simulink library "dspobslib"  (Simulink 8.0)
settings: Solver=ode45  SolverMode=SingleTasking  StartTime=0.0  StopTime=10.0  RelTol=1e-3
values from neighbouring files (symbols this model uses):
  D = D + B    [rebuffer_delay.m]
  ic = eval(icStr)    [dsparch3Transform.m]
undefined symbols (not defined in the file or in its folder): phh, phl
libraries: dspsigattribs x14, dspsigops x5, dspobslib x3, dspmtrx3 x1, dspmathops x1, dspbuff3 x1
settings Model: RequirementInfo=9  Creator=don  LastModifiedBy=amoyer  CovMetricSettings=d  ExtModeAutoUpdateStatusClock=off
settings Model: ForwardingTableString=|
  | ||__slOldName__||dspobslib/Yule-Walker IIR
  | Filter Design||__slNewName__||dspddes3/Yule-Walker IIR
  | Filter Design||__slOldName__||dspobslib/Digital IIR
  | Filter Design||__slNewName__||dspddes3/Digital IIR
  | Filter Design||__slOldName__||dspobslib/Digital FIR Raised
  | Cosine Filter Design||__slNewName__||dspddes3/Digital FIR Raised
  | Cosine Filter Design||__slOldName__||dspobslib/Least Squares FIR
  | Filter Design||__slNewName__||dspddes3/Least Squares FIR
  | Filter Design||__slOldName__||dspobslib/Remez FIR
  | Filter Design||__slNewName__||dspddes3/Remez FIR
  | Filter Design||__slOldName__||dspobslib/Digital FIR
  | Filter Design||__slNewName__||dspddes3/Digital FIR
  | Filter Design||__slOldName__||dspobslib/Time-Varying
  | Lattice Filter||__slNewName__||dsparch3/Time-Varying
  | Lattice Filter||__slOldName__||dspobslib/Time-Varying Direct-
  | Form II Transpose Filter||__slNewName__||dsparch3/Time-Varying Direct-
  | Form II Transpose Filter||__slOldName__||dspobslib/Direct-Form II
  | Transpose Filter||__slNewName__||dsparch3/Direct-Form II
  | Transpose Filter||__slOldName__||dspobslib/Biquadratic
  | Filter||__slNewName__||dsparch4/Biquad Filter

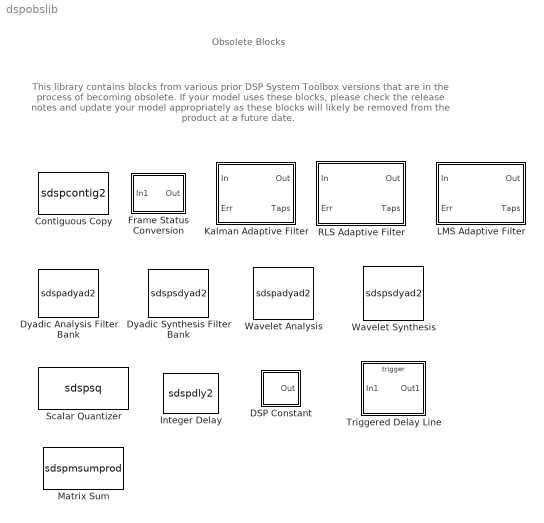
== system dspobslib ==
  note: Obsolete Blocks
  note: This library contains blocks from various prior DSP System Toolbox versions
      | that are in the process of becoming obsolete. If your model uses these blocks, please
      | check the release notes and update your model appropriately as these blocks will likely
      | be removed from the product at a future date.
  Contiguous Copy : S-Function  FunctionName=sdspcontig2  EnableBusSupport=off  mask(Contiguous Copy){}
      mask help: Create a contiguous copy of input data. For use with blocks that only accept contiguous data during simulation or code generation.
      mask Help: eval('blocksethelp');
      mask Display: disp('Contiguous\nCopy');
  DSP Constant : Subsystem  mask(DSP Constant){Value=1, SampleMode=Discrete, discreteOutput=Sample-based, continuousOutput=Sample-based, sampTime=1, framePeriod=2, additionalParams=off, allowOverrides=on, dataType=Inherit from 'Constant value', isSigned=on, wordLen=16, udDataType=sfix(16), fracBitsMode=Best precision, numFracBits=15, InterpretAs1D=-inf, Ts=-inf, FramebasedOutput=-inf}
      mask prompts: Value "Constant value:"; SampleMode "Sample mode:"; discreteOutput "Output:"; continuousOutput "Output:"; sampTime "Sample time:"; framePeriod "Frame period:"; additionalParams "------- Show additional parameters --------"; allowOverrides "Allow overrides from DSP Fixed-Point Attributes blocks"; dataType "Output data type:"; isSigned "Signed"; wordLen "Word length:"; udDataType "User-defined data type:"; fracBitsMode "Set fraction length in output to:"; numFracBits "Fraction length:"; InterpretAs1D "old Interpret as 1D checkbox"; Ts "old Sample time/Frame period"; FramebasedOutput "old Frame-based output checkbox"
      mask help: Output a discrete-time or continuous-time constant.
      mask init:
      | dispValue = get_param(gcbh, 'Value');
      | dspblkdspconst2('init');
      | dspblkdspconst2('update');
      mask Help: eval('blocksethelp');
      mask TypeOptions SampleMode: Discrete | Continuous
      mask Callback SampleMode: dspblkdspconst2;
      mask TypeOptions discreteOutput: Sample-based (interpret vectors as 1-D) | Sample-based | Frame-based
      mask Callback discreteOutput: dspblkdspconst2;
      mask TypeOptions continuousOutput: Sample-based (interpret vectors as 1-D) | Sample-based
      mask Callback continuousOutput: dspblkdspconst2;
      mask TypeOptions dataType: double | single | int8 | uint8 | int16 | uint16 | int32 | uint32 | boolean | Fixed-point | User-defined | Inherit from 'Constant value' | Inherit via back propagation
      mask Callback dataType: dspblkdspconst2;
      mask Callback udDataType: dspblkdspconst2;
      mask TypeOptions fracBitsMode: Best precision | User-defined
      mask Callback fracBitsMode: dspblkdspconst2;
      mask Display: disp(dispValue);
  Dyadic Analysis Filter Bank : S-Function  FunctionName=sdspadyad2  Parameters=phl,phh,numLevels,tree, hl, hh  EnableBusSupport=off  mask(Dyadic Analysis Filter Bank){hl=fir1(12,0.4), hh=fir1(12,0.6,'high'), numLevels=2, tree=Asymmetric}
      mask prompts: hl "Lowpass FIR filter coefficients:"; hh "Highpass FIR filter coefficients:"; numLevels "Number of levels:"; tree "Tree structure:"
      mask help: Apply a sequence of FIR filters to the input signal, downsampling by two following each filtering operation. With reference to the icon on the block, a lowpass filter is applied at each descending branch and a highpass filter is applied at each non-descending branch. Normally, the lowpass and highpass filters are complementary, as in a typical wavelet-based signal decomposition.
      mask init:
      | [phl,phh,x,y,str] = dspblkadyad2(hl,hh,numLevels,tree);
      mask Help: eval('blocksethelp');
      mask TypeOptions tree: Asymmetric | Symmetric
      mask Display:
      | text(0.1,0.15,str)
      | plot(x,y)
  Dyadic Synthesis Filter Bank : S-Function  FunctionName=sdspsdyad2  Parameters=phl,phh,numLevels,tree,hl,hh  EnableBusSupport=off  mask(Dyadic Synthesis Filter Bank){hl=fir1(12,0.4), hh=fir1(12,0.6,'high'), numLevels=2, tree=Asymmetric}
      mask prompts: hl "Lowpass FIR filter coefficients:"; hh "Highpass FIR filter coefficients:"; numLevels "Number of levels:"; tree "Tree structure:"
      mask help: Apply a sequence of FIR filters to the input signals, upsampling by two following each filtering operation. With reference to the icon on the block, a lowpass filter is applied at each descending branch and a highpass filter is applied at each non-descending branch. Normally, the lowpass and highpass filters are complementary, as in a typical wavelet-based signal reconstruction.
      mask init:
      | [phl,phh,x,y,str] = dspblksdyad2(hl,hh,numLevels,tree);
      mask Help: eval('blocksethelp');
      mask TypeOptions tree: Asymmetric | Symmetric
      mask Display:
      | text(0.80,0.15,str)
      | plot(x,y)
  Frame Status Conversion : Subsystem  mask(Frame Status Conversion){growRefPort=off, outframe=Frame-based}
      mask prompts: growRefPort "Inherit output frame status from Ref input port"; outframe "Output signal:"
      mask help: Specify the frame status of the output signal.
      mask init:
      | [p, str] = dspblkfrmconv('init');
      mask Help: eval('blocksethelp');
      mask Callback growRefPort: dspblkfrmconv
      mask TypeOptions outframe: Frame-based | Sample-based
      mask Display:
      | port_label(p.in1,   p.i1,  p.i1s);
      | port_label(p.in2,   p.i2,  p.i2s);
      | port_label(p.out, p.o1, p.o1s);
      | disp(str)
  Integer Delay : S-Function  FunctionName=sdspdly2  Parameters=delay,ic,reset  EnableBusSupport=off  mask(Integer Delay){delay=1, ic=0, reset_popup=None}
      mask prompts: delay "Delay (samples):"; ic "Initial conditions:"; reset_popup "Reset port:"
      mask help: Delay discrete-time input by a fixed integer number of sample periods.
      mask init:
      | delayValue = get_param(gcbh, 'delay');
      | str = dspblkdly2('icon',delayValue,delay);
      | dx = 0.01*length(str);
      | reset = reset_popup-1;
      | if (reset == 0)
      | 	s.i1 = 1; s.i1s = '';
      | 	s.i2 = 1; s.i2s = '';
      | else
      | 	s.i1 = 1; s.i1s = 'In';
      | 	s.i2 = 2; s.i2s = 'Rst';
      | end
      mask Help: eval('blocksethelp');
      mask TypeOptions reset_popup: None | Rising edge | Falling edge | Either edge | Non-zero sample
      mask Display:
      | text(0.42-dx, 0.4, 'z'); text(0.5-dx, 0.6, str);
      | port_label('input',s.i1,s.i1s);
      | port_label('input',s.i2,s.i2s);
  Kalman Adaptive Filter : Subsystem  mask(Kalman Adaptive Filter){Ntaps=64, Jmin=0.3, q=0.1, ic0=0, K0=0.5, Adapt=off, RstPort=None}
      mask prompts: Ntaps "FIR filter length:"; Jmin "Measurement noise variance:"; q "Process noise variance:"; ic0 "Initial value of filter taps:"; K0 "Initial error correlation matrix:"; Adapt "Adapt port"; RstPort "Reset port:"
      mask help:
      | One-step Kalman predictor algorithm for adaptive FIR filtering of input signal.
      |
      | Select the Adapt port check box to create an Adapt port on the block. When the input to this port is nonzero, the block enables filter adaptation. When the input to this port is zero, filter adaptation is disabled.
      |
      | If the Reset port is enabled and a reset event occurs, the block resets the filter weights to their initial values.
      mask init:
      | if prod(size(ic0))==1, ic = ic0(ones(Ntaps,1)); else ic = ic0; end
      | if prod(size(K0))==1, K = K0.*eye(Ntaps);
      | elseif any(size(K0)==1), K = diag(K0);
      | else K=K0; end
      | % ic = ic0;
      | % K = K0;
      | dspblkadpt('init');
      mask Help: eval('blocksethelp');
      mask TypeOptions RstPort: None | Rising edge | Falling edge | Either edge | Non-zero sample
      mask Display: disp('Kalman')
  LMS Adaptive Filter : Subsystem  mask(LMS Adaptive Filter){n=32, mu=.65, ic=0.0, leakage=1.0, normalized=on, Adapt=off, RstPort=None}
      mask prompts: n "FIR filter length:"; mu "Step-size, mu:"; ic "Initial value of filter taps:"; leakage "Leakage factor (0 to 1):"; normalized "Use normalization"; Adapt "Adapt input"; RstPort "Reset input:"
      mask help:
      | Least mean-square (LMS) algorithm for adaptive FIR filtering of input signal.  Energy normalization may optionally be disabled.
      |
      | If 'Adapt input' is checked and the Adapt signal is zero, the algorithm temporarily disables adaptation of the filter coefficients.  A non-zero signal enables filter adaptation.
      |
      | If the 'Reset input' is enabled and the Reset signal transitions appropriately, the filter coefficients are reset to the initial conditions.
      mask init:
      | if normalized, s='nLMS'; else s='LMS'; end
      | dspblkadpt('init');
      mask Help: eval('blocksethelp');
      mask TypeOptions RstPort: None | Rising edge | Falling edge | Either edge | Non-zero sample
      mask Display: disp(s);
  Matrix Sum : S-Function  DialogController=dspDDGCreate  DialogControllerArgs=DataTag3  FunctionName=sdspmsumprod  Parameters=Dim,1,[],[],-1,0,0,-1,0,0,dtInfo.accumMode,dtInfo.accumWordLength,dtInfo.accumFracLength,dtInfo.outputMode,dtInfo.outputWordLength,dtInfo.outputFracLength,dtInfo.roundingMode,dtInfo.overflowMode  EnableBusSupport=off  mask(Matrix Sum){Dim=Columns, additionalParams=off, allowOverrides=on, outputMode=Same as accumulator, outputWordLength=16, outputFracLength=15, accumMode=Inherit via internal rule, accumWordLength=32, accumFracLength=30, roundingMode=Floor, overflowMode=off, LockScale=off}
      mask prompts: Dim "Sum over:"; additionalParams "------- Show additional parameters -------"; allowOverrides "Allow overrides from DSP Fixed-Point Attributes blocks"; outputMode "Fixed-point output attributes:"; outputWordLength "Output word length:"; outputFracLength "Output fraction length:"; accumMode "Fixed-point accumulator attributes:"; accumWordLength "Accumulator word length:"; accumFracLength "Accumulator fraction length:"; roundingMode "Round integer calculations toward:"; overflowMode "Saturate on integer overflow"; LockScale "Lock scaling"
      mask help: Sum the elements of a matrix along its rows, its columns, or over all its elements. Note that 1-D input signals produce a single scalar output equal to the sum of the individual elements.
      mask init:
      | if (Dim==1), str='Row\nSum';
      | elseif (Dim==2), str='Column\nSum';
      | else str='Sum of\nAll Elements';
      | end
      | 
      | %misc       1 USED
      | %output     2 USED
      | %accum      4 USED
      | dtInfo = dspGetFixptDataTypeInfo(gcbh,7);
      mask Help: eval('blocksethelp');
      mask TypeOptions Dim: Rows | Columns | Entire input
      mask TypeOptions outputMode: Same as accumulator | Same as input | Binary point scaling | Slope and bias scaling | User-defined
      mask TypeOptions accumMode: Inherit via internal rule | Same as input | Binary point scaling | Slope and bias scaling | User-defined
      mask TypeOptions roundingMode: Ceiling | Convergent | Floor | Nearest | Round | Simplest | Zero
      mask Display: disp(str);
  RLS Adaptive Filter : Subsystem  mask(RLS Adaptive Filter){Ntaps=32, Lambda=1.0, ic=0.0, phi0=0.1, Adapt=off, RstPort=None}
      mask prompts: Ntaps "FIR filter length:"; Lambda "Memory weighting factor (0 to 1):"; ic "Initial value of filter taps:"; phi0 "Initial input variance estimate:"; Adapt "Adapt input"; RstPort "Reset input:"
      mask help:
      | Exponentially weighted recursive least-squares (RLS) algorithm for adaptive FIR filtering of input signal.
      |
      | If 'Adapt input' is checked and the Adapt signal is zero, the algorithm temporarily disables adaptation of the filter coefficients.  A non-zero signal enables filter adaptation.
      |
      | If the 'Reset input' is enabled and the Reset signal transitions appropriately, the filter coefficients are reset to the initial conditions.
      mask init:
      | dspblkadpt('init');
      mask Help: eval('blocksethelp');
      mask TypeOptions RstPort: None | Rising edge | Falling edge | Either edge | Non-zero sample
      mask Display: disp('RLS')
  Scalar Quantizer : S-Function  FunctionName=sdspsq  Parameters=Qmode,QparamSource,partitionUnBound,codebook,SearchMethod,tieBreakRule,outQError, invalidin, dtype, idtype, cwdtype,1,1  EnableBusSupport=off  mask(Scalar Quantizer){Qmode=Encoder, QparamSource=Specify via dialog, partitionUnBound=[   0  1  2  3  4  5    6  7  8    9], codebook=[0.0    1.5     2.5    3.5    4.5   5.5   6.5  7.5  8.5 ], SearchMethod=Binary, tieBreakRule=Choose the lower index, outQError=off, invalidin=Clip and warn, dtype=off, idtype=int32, cwdtype=double}
      mask prompts: Qmode "Quantizer mode:"; QparamSource "Source of quantizer parameters:"; partitionUnBound "Boundary points:"; SearchMethod "Searching method:"; tieBreakRule "Tie-breaking rule:"; outQError "Output the quantization error"; invalidin "Action for out of range input:"; dtype "--------------- Show additional parameters ---------------"; idtype "Output index data type:"; cwdtype "Output data type:"
      mask help:
      | The Scalar Quantizer block has three modes of operation.
      | In Encoder mode, the block maps each input value to a quantization region by comparing the input value to the user-specified quantizer boundary points. The block outputs the index of the associated region.
      | In Decoder mode, the block transforms the input index values into quantized output values, defined by the quantizer codebook.
      | In the Encoder & Decoder mode, the block performs both the encoding and decoding operations. The block outputs the index values and the quantized output values.
      |
      | The Boundary points parameter is a vector of dimension N whose values are arranged in ascending order ([p1 p2 ... pN]). The quantizer codebook is a vector of length (N-1). The quantizer is unbounded if p1 is -inf and pN is inf. When the quantizer is bounded, p1 is the lower bound for the input values. Any input less than p1 is clipped to p1 and then quantized. Similarly, pN is the upper bound for the input values. Any input greater than pN is clipped to pN and is then quantized.
      mask init:
      | [si,so,disp_str]=dspblksq('icon');
      mask Help: eval('blocksethelp');
      mask TypeOptions Qmode: Encoder | Decoder | Encoder and decoder
      mask Callback Qmode: dspblksq
      mask TypeOptions QparamSource: Specify via dialog | Input ports
      mask Callback QparamSource: dspblksq
      mask TypeOptions SearchMethod: Linear | Binary
      mask TypeOptions tieBreakRule: Choose the lower index | Choose the higher index
      mask TypeOptions invalidin: Clip | Clip and warn | Error
      mask Callback invalidin: dspblksq
      mask Callback dtype: dspblksq
      mask TypeOptions idtype: int8 | uint8 | int16 | uint16 | int32 | uint32
      mask TypeOptions cwdtype: double | single | int8 | uint8 | int16 | uint16 | int32 | uint32
      mask Display:
      | disp(disp_str);
      | port_label('input',si(1).port, si(1).txt);
      | port_label('input',si(2).port, si(2).txt);
      | port_label('input',si(3).port, si(3).txt);
      | port_label('output',so(1).port, so(1).txt);
      | port_label('output',so(2).port, so(2).txt);
      | port_label('output',so(3).port, so(3).txt);
  Triggered Delay Line : Subsystem  TreatAsAtomicUnit=on  mask(Triggered Delay Line){trig=Rising edge, siz=64, ic=0, TreatMby1Signals=One channel}
      mask prompts: trig "Trigger type:"; siz "Delay line size:"; ic "Initial conditions:"; TreatMby1Signals "Treat Mx1 and unoriented sample-based signals as:"
      mask help: Shift out delay line contents and store input data into start of delay line when trigger event occurs.
      mask init:
      | switch trig
      | case 1, s='rising';
      | case 2, s='falling';
      | case 3, s='either';
      | end
      | set_param([gcb '/Trigger'],'triggertype',s);
      | 
      | blkh = gcbh;
      | blkUserData = get_param(blkh, 'UserData');
      | if ~isfield(blkUserData, 'hasMChanOption')
      |     % Create and save the UserData field
      |     blkUserData.hasMChanOption = true;
      |     set_param(blkh, 'UserDataPersistent', 'on', ...
      |     'UserData', blkUserData);
      |     set_param(blkh, 'TreatMby1Signals', ...
      |     'M channels (this choice will be removed - see release notes)');
      | end
      | 
      | treat = get_param(blkh, 'TreatMby1Signals');
      | set_param([gcb '/Delay Line'], 'TreatMby1Signals', treat);
      mask Help: eval('blocksethelp');
      mask TypeOptions trig: Rising edge | Falling edge | Either edge
      mask TypeOptions TreatMby1Signals: One channel | M channels (this choice will be removed - see release notes)
      mask Display: disp('Delay\nLine');
  Wavelet Analysis : S-Function  FunctionName=sdspadyad2  Parameters=phl, phh, NumLevels, tree, hl, hh  EnableBusSupport=off  mask(Wavelet Analysis){Wname=Haar, OrdRec_ordDec=[1 / 1], Order=2, NumLevels=2}
      mask prompts: Wname "Wavelet name:"; OrdRec_ordDec "Filter order [synthesis / analysis]:"; Order "Wavelet order:"; NumLevels "Number of levels:"
      mask help:
      | Multilevel discrete 1-D wavelet decomposition using a specific wavelet.
      |
      | The Wavelet Toolbox must be installed to use this block.
      mask init:
      | [x,y,str] = dspblkwavedec2('icon');
      | [phl, phh, tree, hl, hh] = dspblkwavedec2('init');
      mask Help: eval('blocksethelp');
      mask TypeOptions Wname: Haar | Daubechies | Symlets | Coiflets | Biorthogonal | Reverse Biorthogonal | Discrete Meyer
      mask Callback Wname: dspblkwavedec2
      mask TypeOptions OrdRec_ordDec: [1 / 1] | [1 / 3] | [1 / 5] | [2 / 2] | [2 / 4] | [2 / 6] | [2 / 8] | [3 / 1] | [3 / 3] | [3 / 5] | [3 / 7] | [3 / 9] | [4 / 4] | [5 / 5] | [6 / 8]
      mask Display:
      | text(0.08,0.1,str)
      | plot(x,y)
  Wavelet Synthesis : S-Function  FunctionName=sdspsdyad2  Parameters=phl, phh, NumLevels, tree, hl, hh  EnableBusSupport=off  mask(Wavelet Synthesis){Wname=Haar, OrdRec_ordDec=[1 / 1], Order=2, NumLevels=2}
      mask prompts: Wname "Wavelet name:"; OrdRec_ordDec "Filter order [synthesis, analysis]:"; Order "Wavelet order:"; NumLevels "Number of levels:"
      mask help:
      | Multilevel discrete 1-D wavelet reconstruction using a specific wavelet.
      |
      | The Wavelet Toolbox must be installed to use this block.
      mask init:
      | [x,y,str] = dspblkwaverec2('icon');
      | [phl, phh, tree, hl, hh] = dspblkwaverec2('init');
      mask Help: eval('blocksethelp');
      mask TypeOptions Wname: Haar | Daubechies | Symlets | Coiflets | Biorthogonal | Reverse Biorthogonal | Discrete Meyer
      mask Callback Wname: dspblkwaverec2
      mask TypeOptions OrdRec_ordDec: [1 / 1] | [1 / 3] | [1 / 5] | [2 / 2] | [2 / 4] | [2 / 6] | [2 / 8] | [3 / 1] | [3 / 3] | [3 / 5] | [3 / 7] | [3 / 9] | [4 / 4] | [5 / 5] | [6 / 8]
      mask Display:
      | text(0.37,0.15,str)
      | plot(x,y)

== system dspobslib/DSP Constant ==
  Constant : Constant  Value=Value  VectorParams1D=off  SampleTime=sampTime
  Frame Status Conversion : FrameConversion  OutFrame=Sample-based
  Out : Outport
  wires:
  Constant/1 -> Frame Status Conversion/1
  Frame Status Conversion/1 -> Out/1

== system dspobslib/Frame Status Conversion ==
  In1 : Inport
  Frame Status : FrameConversion
  Out : Outport
  wires:
  In1/1 -> Frame Status/1
  Frame Status/1 -> Out/1

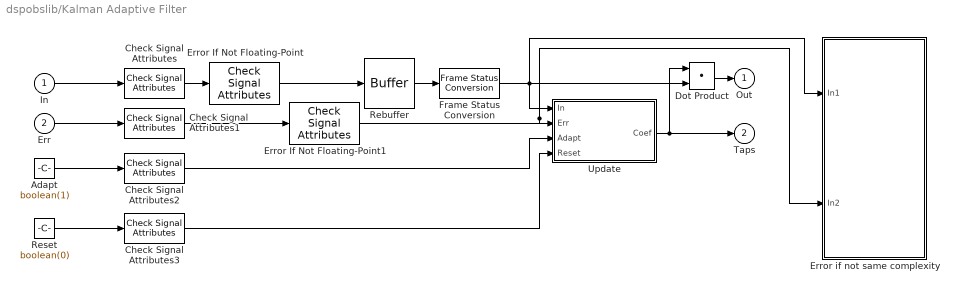
== system dspobslib/Kalman Adaptive Filter ==
  In : Inport
  Err : Inport  Port=2
  Adapt : Constant  Value=boolean(1)
  Check Signal Attributes{,1..3} (4 alike) : dspsigattribs/Check Signal Attributes  SystemSampleTime=-1  SigAttribCheckMethod=Does not match attributes exactly  Complexity=Ignore  Frame=Sample-based  DimsCheckMethod=Is...  Dimensions=Scalar (1-D or 2-D)  DatatypeCheckMethod=Ignore  DatatypeGeneral=Boolean  DtypeFloatSpecific=Any floating-point  DtypeFixedSpecific=Any fixed-point  DtypeIntSpecific=Any integer  SampleMode=Ignore
  Dot Product : DotProduct  OutDataTypeStr=Inherit: Inherit via internal rule
  Error If Not Floating-Point : dspsigattribs/Check Signal Attributes  SystemSampleTime=-1  SigAttribCheckMethod=Does not match attributes exactly  Complexity=Ignore  Frame=Ignore  DimsCheckMethod=Ignore  Dimensions=1-D  DatatypeCheckMethod=Is...  DatatypeGeneral=Floating-point  DtypeFloatSpecific=Any floating-point  DtypeFixedSpecific=Any fixed-point  DtypeIntSpecific=Any integer  SampleMode=Ignore
  Error If Not Floating-Point1 : dspsigattribs/Check Signal Attributes  SystemSampleTime=-1  SigAttribCheckMethod=Does not match attributes exactly  Complexity=Ignore  Frame=Ignore  DimsCheckMethod=Ignore  Dimensions=1-D  DatatypeCheckMethod=Is...  DatatypeGeneral=Floating-point  DtypeFloatSpecific=Any floating-point  DtypeFixedSpecific=Any fixed-point  DtypeIntSpecific=Any integer  SampleMode=Ignore
  Error if not same complexity : Subsystem  TreatAsAtomicUnit=on  SimViewingDevice=on
  Frame Status Conversion : dspobslib/Frame Status Conversion  SystemSampleTime=-1  growRefPort=off  outframe=Sample-based
  Rebuffer : Buffer  N=Ntaps  V=Ntaps-1  TreatMby1Signals=One channel
  Reset : Constant  Value=boolean(0)
  Update : Subsystem
  Out : Outport  InitialOutput=0
  Taps : Outport  Port=2  InitialOutput=0
  wires:
  Err/1 -> Check Signal Attributes1/1
  In/1 -> Check Signal Attributes/1
  Adapt/1 -> Check Signal Attributes2/1
  Dot Product/1 -> Out/1
  Rebuffer/1 -> Frame Status Conversion/1
  Update/1(Coef) -> Taps/1, Dot Product/1
  Check Signal Attributes1/1 -> Error If Not Floating-Point1/1
  Check Signal Attributes/1 -> Error If Not Floating-Point/1
  Check Signal Attributes2/1 -> Update/3(Adapt)
  Frame Status Conversion/1 -> Update/1(In), Dot Product/2, Error if not same complexity/1(In1)
  Reset/1 -> Check Signal Attributes3/1
  Check Signal Attributes3/1 -> Update/4(Reset)
  Error If Not Floating-Point/1 -> Rebuffer/1
  Error If Not Floating-Point1/1 -> Error if not same complexity/2(In2), Update/2(Err)

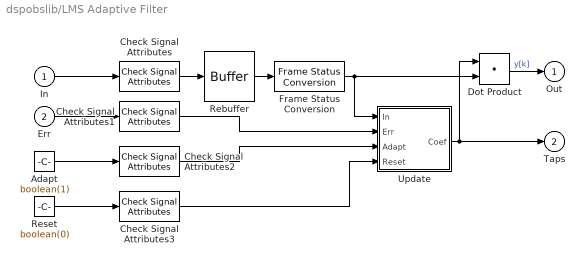
== system dspobslib/LMS Adaptive Filter ==
  In : Inport
  Err : Inport  Port=2
  Adapt : Constant  Value=boolean(1)
  Check Signal Attributes{,1..3} (4 alike) : dspsigattribs/Check Signal Attributes  SigAttribCheckMethod=Does not match attributes exactly  Complexity=Ignore  Frame=Sample-based  DimsCheckMethod=Is...  Dimensions=Scalar (1-D or 2-D)  DatatypeCheckMethod=Ignore  DatatypeGeneral=Boolean  DtypeFloatSpecific=Any floating-point  DtypeFixedSpecific=Any fixed-point  DtypeIntSpecific=Any integer  SampleMode=Ignore
  Dot Product : DotProduct  InputSameDT=on  OutDataTypeStr=Inherit: Inherit via internal rule
  Frame Status Conversion : dspobslib/Frame Status Conversion  growRefPort=off  outframe=Sample-based
  Rebuffer : Buffer  N=n  V=n-1  TreatMby1Signals=One channel
  Reset : Constant  Value=boolean(0)
  Update : Subsystem
  Out : Outport  InitialOutput=0
  Taps : Outport  Port=2  InitialOutput=0
  wires:
  Dot Product/1 -> Out/1  "y[k]"
  Update/1(Coef) -> Taps/1, Dot Product/1
  Rebuffer/1 -> Frame Status Conversion/1
  In/1 -> Check Signal Attributes/1
  Check Signal Attributes/1 -> Rebuffer/1
  Err/1 -> Check Signal Attributes1/1
  Check Signal Attributes1/1 -> Update/2(Err)
  Adapt/1 -> Check Signal Attributes2/1
  Check Signal Attributes2/1 -> Update/3(Adapt)
  Frame Status Conversion/1 -> Update/1(In), Dot Product/2
  Reset/1 -> Check Signal Attributes3/1
  Check Signal Attributes3/1 -> Update/4(Reset)

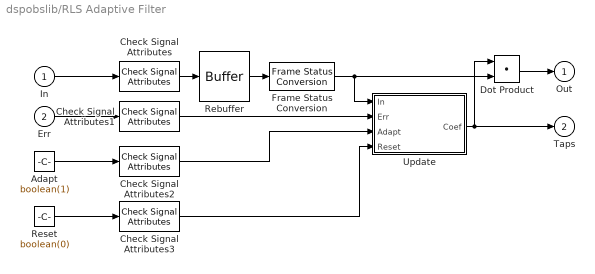
== system dspobslib/RLS Adaptive Filter ==
  In : Inport
  Err : Inport  Port=2
  Adapt : Constant  Value=boolean(1)
  Check Signal Attributes{,1..3} (4 alike) : dspsigattribs/Check Signal Attributes  SigAttribCheckMethod=Does not match attributes exactly  Complexity=Ignore  Frame=Sample-based  DimsCheckMethod=Is...  Dimensions=Scalar (1-D or 2-D)  DatatypeCheckMethod=Ignore  DatatypeGeneral=Boolean  DtypeFloatSpecific=Any floating-point  DtypeFixedSpecific=Any fixed-point  DtypeIntSpecific=Any integer  SampleMode=Ignore
  Dot Product : DotProduct  InputSameDT=on  OutDataTypeStr=Inherit: Inherit via internal rule
  Frame Status Conversion : dspobslib/Frame Status Conversion  growRefPort=off  outframe=Sample-based
  Rebuffer : Buffer  N=Ntaps  V=Ntaps-1  TreatMby1Signals=One channel
  Reset : Constant  Value=boolean(0)
  Update : Subsystem
  Out : Outport  InitialOutput=0
  Taps : Outport  Port=2  InitialOutput=0
  wires:
  Dot Product/1 -> Out/1
  Update/1(Coef) -> Taps/1, Dot Product/1
  Rebuffer/1 -> Frame Status Conversion/1
  In/1 -> Check Signal Attributes/1
  Check Signal Attributes/1 -> Rebuffer/1
  Err/1 -> Check Signal Attributes1/1
  Check Signal Attributes1/1 -> Update/2(Err)
  Adapt/1 -> Check Signal Attributes2/1
  Check Signal Attributes2/1 -> Update/3(Adapt)
  Frame Status Conversion/1 -> Update/1(In), Dot Product/2
  Reset/1 -> Check Signal Attributes3/1
  Check Signal Attributes3/1 -> Update/4(Reset)

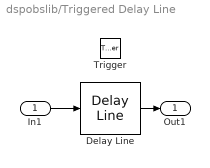
== system dspobslib/Triggered Delay Line ==
  In1 : Inport
  Trigger : TriggerPort  ZeroCross=off
  Delay Line : dspbuff3/Delay Line  siz=siz  ic=ic  directfeed=off  enable_output=off  hold_output=off  TreatMby1Signals=One channel
  Out1 : Outport  InitialOutput=ic
  wires:
  In1/1 -> Delay Line/1
  Delay Line/1 -> Out1/1

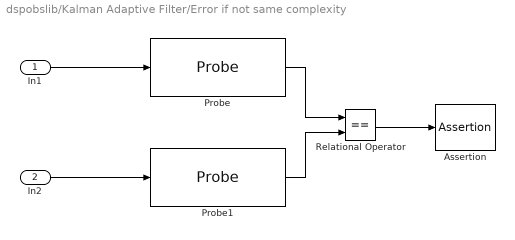
== system dspobslib/Kalman Adaptive Filter/Error if not same complexity ==
  In1 : Inport
  In2 : Inport  Port=2
  Assertion : Assertion  Enabled=on  AssertionFailFcn=error('The signals connected to the Input and Error ports of the Kalman Adaptive Filter block must have the same complexity.')
  Probe : Probe  ProbeWidth=off  ProbeSampleTime=off  ProbeComplexityDataType=boolean
  Probe1 : Probe  ProbeWidth=off  ProbeSampleTime=off  ProbeComplexityDataType=boolean
  Relational Operator : RelationalOperator  Operator===  OutDataTypeStr=boolean  ZeroCross=off  InputSameDT=on
  wires:
  Probe/1 -> Relational Operator/1
  Probe1/1 -> Relational Operator/2
  In1/1 -> Probe/1
  In2/1 -> Probe1/1
  Relational Operator/1 -> Assertion/1

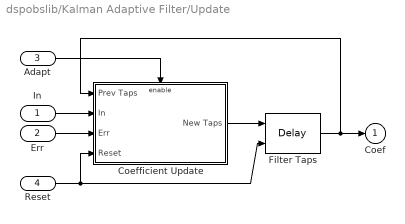
== system dspobslib/Kalman Adaptive Filter/Update ==
  In : Inport
  Err : Inport  Port=2
  Adapt : Inport  Port=3
  Reset : Inport  Port=4
  Coefficient Update : Subsystem  TreatAsAtomicUnit=on
  Filter Taps : dspsigops/Delay  dly_unit=Samples  delay=1  ic_detail=off  dif_ic_for_ch=on  dif_ic_for_dly=off  ic=ic  reset_popup=Non-zero sample
  Coef : Outport  InitialOutput=0
  wires:
  Filter Taps/1 -> Coef/1, Coefficient Update/1(Prev Taps)
  Coefficient Update/1(New Taps) -> Filter Taps/1
  In/1 -> Coefficient Update/2(In)
  Err/1 -> Coefficient Update/3(Err)
  Adapt/1 -> Coefficient Update/Enable
  Reset/1 -> Coefficient Update/4(Reset), Filter Taps/2

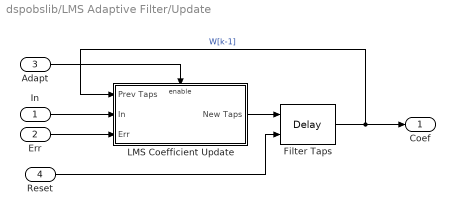
== system dspobslib/LMS Adaptive Filter/Update ==
  In : Inport
  Err : Inport  Port=2
  Adapt : Inport  Port=3
  Reset : Inport  Port=4
  Filter Taps : dspsigops/Delay  dly_unit=Samples  delay=1  ic_detail=off  dif_ic_for_ch=off  dif_ic_for_dly=off  ic=ic  reset_popup=Non-zero sample
  LMS Coefficient Update : Subsystem  TreatAsAtomicUnit=on
  Coef : Outport  InitialOutput=0
  wires:
  LMS Coefficient Update/1(New Taps) -> Filter Taps/1
  Err/1 -> LMS Coefficient Update/3(Err)
  In/1 -> LMS Coefficient Update/2(In)
  Filter Taps/1 -> Coef/1, LMS Coefficient Update/1(Prev Taps)  "W[k-1]"
  Adapt/1 -> LMS Coefficient Update/Enable
  Reset/1 -> Filter Taps/2

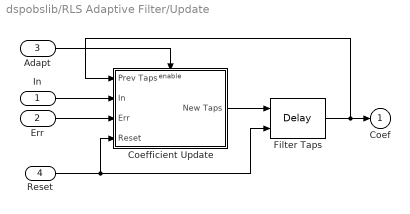
== system dspobslib/RLS Adaptive Filter/Update ==
  In : Inport
  Err : Inport  Port=2
  Adapt : Inport  Port=3
  Reset : Inport  Port=4
  Coefficient Update : Subsystem  TreatAsAtomicUnit=on
  Filter Taps : dspsigops/Delay  dly_unit=Samples  delay=1  ic_detail=off  dif_ic_for_ch=off  dif_ic_for_dly=off  ic=ic  reset_popup=Non-zero sample
  Coef : Outport  InitialOutput=0
  wires:
  Err/1 -> Coefficient Update/3(Err)
  Filter Taps/1 -> Coef/1, Coefficient Update/1(Prev Taps)
  Coefficient Update/1(New Taps) -> Filter Taps/1
  In/1 -> Coefficient Update/2(In)
  Adapt/1 -> Coefficient Update/Enable
  Reset/1 -> Coefficient Update/4(Reset), Filter Taps/2

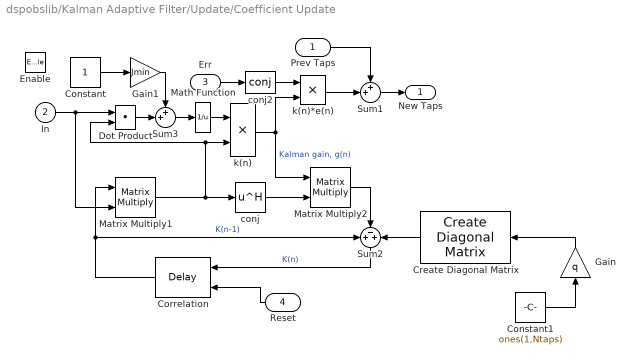
== system dspobslib/Kalman Adaptive Filter/Update/Coefficient Update ==
  Prev Taps : Inport
  In : Inport  Port=2
  Err : Inport  Port=3
  Reset : Inport  Port=4
  Enable : EnablePort  PropagateVarSize=During execution  ZeroCross=off
  Constant : Constant  OutDataTypeStr=Inherit: Inherit via back propagation
  Constant1 : Constant  Value=ones(1,Ntaps)  OutDataTypeStr=Inherit: Inherit via back propagation
  Correlation : dspsigops/Delay  dly_unit=Samples  delay=1  ic_detail=off  dif_ic_for_ch=on  dif_ic_for_dly=off  ic=K  reset_popup=Either edge
  Create Diagonal Matrix : dspmtrx3/Create Diagonal Matrix
  Dot Product : DotProduct  InputSameDT=on  OutDataTypeStr=Inherit: Inherit via internal rule
  Gain : Gain  Gain=q  SaturateOnIntegerOverflow=on  OutDataTypeStr=Inherit: Same as input  ParamDataTypeStr=Inherit: Same as input
  Gain1 : Gain  Gain=Jmin  SaturateOnIntegerOverflow=on  OutDataTypeStr=Inherit: Same as input  ParamDataTypeStr=Inherit: Same as input
  Math Function : Math  Operator=reciprocal  SaturateOnIntegerOverflow=on
  Matrix Multiply1 : Product  Multiplication=Matrix(*)
  Matrix Multiply2 : Product  Multiplication=Matrix(*)
  Sum1 : Sum  Inputs=++|  SaturateOnIntegerOverflow=on  InputSameDT=on  OutDataTypeStr=Inherit: Same as first input
  Sum2 : Sum  Inputs=+-+  SaturateOnIntegerOverflow=on  InputSameDT=on  OutDataTypeStr=Inherit: Same as first input
  Sum3 : Sum  Inputs=++|  SaturateOnIntegerOverflow=on  InputSameDT=on  OutDataTypeStr=Inherit: Same as first input
  conj : Math  Operator=hermitian  SaturateOnIntegerOverflow=on
  conj2 : Math  Operator=conj  SaturateOnIntegerOverflow=on
  k(n) : Product  SaturateOnIntegerOverflow=on  InputSameDT=on  OutDataTypeStr=Inherit: Same as first input
  k(n)*e(n) : Product  SaturateOnIntegerOverflow=on  InputSameDT=on  OutDataTypeStr=Inherit: Same as first input
  New Taps : Outport  InitialOutput=ic
  wires:
  Gain1/1 -> Sum3/1
  Gain/1 -> Create Diagonal Matrix/1
  In/1 -> Matrix Multiply1/2, Dot Product/1
  Create Diagonal Matrix/1 -> Sum2/3
  Sum2/1 -> Correlation/1  "K(n)"
  Correlation/1 -> Sum2/1, Matrix Multiply1/1  "K(n-1)"
  Constant/1 -> Gain1/1
  Dot Product/1 -> Sum3/2
  Matrix Multiply2/1 -> Sum2/2
  conj/1 -> Matrix Multiply2/2
  Matrix Multiply1/1 -> conj/1, k(n)/2, Dot Product/2
  Sum3/1 -> Math Function/1
  k(n)/1 -> Matrix Multiply2/1, k(n)*e(n)/2  "Kalman gain, g(n)"
  Err/1 -> conj2/1
  conj2/1 -> k(n)*e(n)/1
  k(n)*e(n)/1 -> Sum1/2
  Prev Taps/1 -> Sum1/1
  Sum1/1 -> New Taps/1
  Math Function/1 -> k(n)/1
  Constant1/1 -> Gain/1
  Reset/1 -> Correlation/2

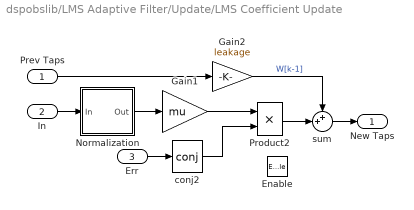
== system dspobslib/LMS Adaptive Filter/Update/LMS Coefficient Update ==
  Prev Taps : Inport
  In : Inport  Port=2
  Err : Inport  Port=3
  Enable : EnablePort  PropagateVarSize=During execution  ZeroCross=off
  Gain1 : Gain  Gain=mu  SaturateOnIntegerOverflow=on  OutDataTypeStr=Inherit: Same as input  ParamDataTypeStr=Inherit: Same as input
  Gain2 : Gain  Gain=leakage  SaturateOnIntegerOverflow=on  OutDataTypeStr=Inherit: Same as input  ParamDataTypeStr=Inherit: Same as input
  Normalization : Subsystem  mask(Replaceable Contents){oname=Normalization, osrc=dspmathops/Normalization, oargs={'NormType','Squared 2-norm','Bias','1e-10'}, replace=~normalized}
      mask prompts: oname "Relative name of blocks to replace:"; osrc "Simulink path to each source block:"; oargs "Parameter/value pairs to each block:"; replace "Replace with short-circuit:"
      mask help: Configurable subsystem holding blocks which may be replaced by virtual short-circuits (muxes) when not needed.
      mask init:
      | opts.name = oname; opts.src = osrc; opts.args = oargs;
      | dspskipblk(gcb,opts,replace);
  Product2 : Product  SaturateOnIntegerOverflow=on  InputSameDT=on  OutDataTypeStr=Inherit: Same as first input
  conj2 : Math  Operator=conj  SaturateOnIntegerOverflow=on
  sum : Sum  Inputs=++|  SaturateOnIntegerOverflow=on  InputSameDT=on  OutDataTypeStr=Inherit: Same as first input
  New Taps : Outport  InitialOutput=ic
  wires:
  conj2/1 -> Product2/2
  Gain1/1 -> Product2/1
  Normalization/1(Out) -> Gain1/1
  Product2/1 -> sum/2
  Gain2/1 -> sum/1  "W[k-1]"
  Prev Taps/1 -> Gain2/1
  In/1 -> Normalization/1(In)
  sum/1 -> New Taps/1
  Err/1 -> conj2/1

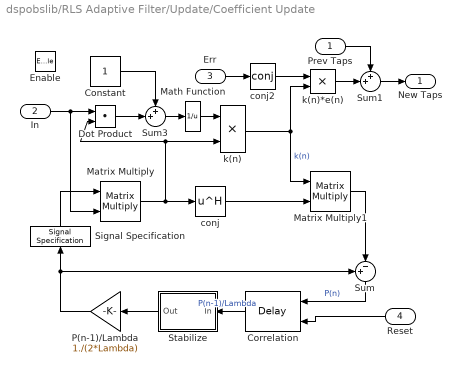
== system dspobslib/RLS Adaptive Filter/Update/Coefficient Update ==
  Prev Taps : Inport
  In : Inport  Port=2
  Err : Inport  Port=3
  Reset : Inport  Port=4
  Enable : EnablePort  PropagateVarSize=During execution  ZeroCross=off
  Constant : Constant  OutDataTypeStr=Inherit: Inherit via back propagation
  Correlation : dspsigops/Delay  dly_unit=Samples  delay=1  ic_detail=off  dif_ic_for_ch=on  dif_ic_for_dly=off  ic=eye(Ntaps)./phi0  reset_popup=Either edge
  Dot Product : DotProduct  InputSameDT=on  OutDataTypeStr=Inherit: Inherit via internal rule
  Math Function : Math  Operator=reciprocal  SaturateOnIntegerOverflow=on
  Matrix Multiply : Product  Multiplication=Matrix(*)
  Matrix Multiply1 : Product  Multiplication=Matrix(*)
  P(n-1)/Lambda : Gain  Gain=1./(2*Lambda)  SaturateOnIntegerOverflow=on  OutDataTypeStr=Inherit: Same as input  ParamDataTypeStr=Inherit: Same as input
  Signal Specification : SignalSpecification  Dimensions=[Ntaps Ntaps]
  Stabilize : Subsystem
  Sum : Sum  Inputs=+-|  SaturateOnIntegerOverflow=on  InputSameDT=on  OutDataTypeStr=Inherit: Same as first input
  Sum1 : Sum  Inputs=++|  SaturateOnIntegerOverflow=on  InputSameDT=on  OutDataTypeStr=Inherit: Same as first input
  Sum3 : Sum  Inputs=++|  SaturateOnIntegerOverflow=on  InputSameDT=on  OutDataTypeStr=Inherit: Same as first input
  conj : Math  Operator=hermitian  SaturateOnIntegerOverflow=on
  conj2 : Math  Operator=conj  SaturateOnIntegerOverflow=on
  k(n) : Product  SaturateOnIntegerOverflow=on  InputSameDT=on  OutDataTypeStr=Inherit: Same as first input
  k(n)*e(n) : Product  SaturateOnIntegerOverflow=on  InputSameDT=on  OutDataTypeStr=Inherit: Same as first input
  New Taps : Outport  InitialOutput=ic
  wires:
  k(n)*e(n)/1 -> Sum1/2
  Constant/1 -> Sum3/1
  Dot Product/1 -> Sum3/2
  In/1 -> Dot Product/1, Matrix Multiply/2
  Sum3/1 -> Math Function/1
  Matrix Multiply/1 -> Dot Product/2, k(n)/2, conj/1
  conj/1 -> Matrix Multiply1/2
  Matrix Multiply1/1 -> Sum/2
  Sum/1 -> Correlation/1  "P(n)"
  k(n)/1 -> Matrix Multiply1/1, k(n)*e(n)/2  "k(n)"
  conj2/1 -> k(n)*e(n)/1
  Prev Taps/1 -> Sum1/1
  Err/1 -> conj2/1
  Sum1/1 -> New Taps/1
  Stabilize/1(Out) -> P(n-1)/Lambda/1
  P(n-1)/Lambda/1 -> Sum/1, Signal Specification/1
  Signal Specification/1 -> Matrix Multiply/1
  Math Function/1 -> k(n)/1
  Correlation/1 -> Stabilize/1(In)  "P(n-1)/Lambda"
  Reset/1 -> Correlation/2

== system dspobslib/LMS Adaptive Filter/Update/LMS Coefficient Update/Normalization ==
  In : Inport
  Normalization : dspmathops/Normalization  NormType=Squared 2-norm  Bias=1e-10
  Out : Outport  InitialOutput=0
  wires:
  In/1 -> Normalization/1
  Normalization/1 -> Out/1

== system dspobslib/RLS Adaptive Filter/Update/Coefficient Update/Stabilize ==
  In : Inport
  Sum2 : Sum  Inputs=|++  SaturateOnIntegerOverflow=on  InputSameDT=on  OutDataTypeStr=Inherit: Same as first input
  conj1 : Math  Operator=hermitian  SaturateOnIntegerOverflow=on
  Out : Outport
  wires:
  In/1 -> conj1/1, Sum2/2  "P(n-1)/Lambda"
  conj1/1 -> Sum2/1
  Sum2/1 -> Out/1
